simulink model "qarm_quick_start_model_virtual"  (R2020a)
settings: Solver=ode4  StartTime=0.0  StopTime=Inf  FixedStep=1/500  RelTol=1e-3
undefined symbols (not defined in the file): HIL
libraries: quarc_library x7, simulink_extras x2
settings Model: ExtModeTrigDuration=10000  Creator=fvranes  LastModifiedBy=mbohra
settings DebuggingCC: UnderspecifiedInitializationDetection=Classic  MergeDetectMultiDrivingBlocksExec=none
settings ModelReferenceCC: PropagateSignalLabelsOutOfModel=off
settings SFSimCC: CustomCodeUndefinedFunction=UseInterfaceOnly

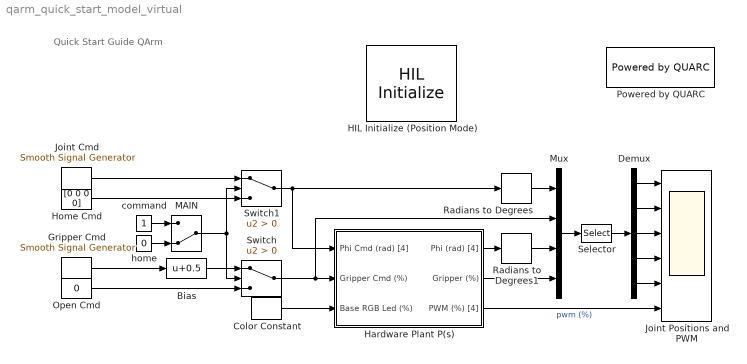
== system qarm_quick_start_model_virtual ==
  note: Quick Start Guide
      | QArm
  Bias : Bias  Bias=0.5
  Color Constant : quarc_library/Sources/Signals/Color Constant  color=[0 1 0]
      settings: SourceProductName=QUARC Targets
  Demux : Demux  Outputs=[2 2 2 2 2]
  Gripper Cmd : quarc_library/Sources/Signals/Smooth Signal Generator  signal_type=Square  source=Internal (dialog parameters)  amplitude=0.5  frequency=0.25  initial_phase=0  sample_time=qc_get_step_size  output_cos=off
      settings: SourceProductName=QUARC Targets
  HIL Initialize (Position Mode) : quarc_library/Data Acquisition/Generic/Configuration/HIL Initialize  object_name=HIL-1  board_type=qarm_usb  board_number=0@tcpip://localhost:18900?nagle='off'  board_options=j0_mode=0;j1_mode=0;j2_mode=0;j3_mode=0;gripper_mode=0;  exclusive=off  active=on  hardware_clocks=[0]  clock_modes=[]  initial_clock_frequencies=[]  set_clock_params_at_start=off  set_clock_params_at_switch_in=off  set_clock_frequencies_at_start=off  set_clock_frequencies_at_switch_in=off  analog_input_channels=[5:9]  analog_input_configurations=[]  analog_input_maximums=[]  analog_input_minimums=[]  set_analog_input_params_at_start=off  set_analog_input_params_at_switch_in=off  analog_output_channels=[]  analog_output_maximums=inf  analog_output_minimums=-inf  initial_analog_outputs=[0]  final_analog_outputs=[0]  watchdog_analog_outputs=[]  set_analog_output_params_at_start=off  set_analog_output_params_at_switch_in=off  set_analog_outputs_at_start=off  set_analog_outputs_at_switch_in=off  set_analog_outputs_at_terminate=off  set_analog_outputs_at_switch_out=off  set_analog_outputs_on_watchdog=off  digital_input_channels=[]  digital_output_channels=[]  digital_output_configuration=[]  initial_digital_outputs=[0]  final_digital_outputs=[0]  watchdog_digital_outputs=[0]  set_digital_output_params_at_start=off  set_digital_output_params_at_switch_in=off  set_digital_outputs_at_start=off  set_digital_outputs_at_switch_in=off  set_digital_outputs_at_terminate=off  set_digital_outputs_at_switch_out=off  set_digital_outputs_on_watchdog=off  encoder_channels=[]  quadrature=[]  encoder_filter_frequency=[]  initial_encoder_counts=[]  set_encoder_params_at_start=off  set_encoder_params_at_switch_in=off  set_encoder_counts_at_start=off  set_encoder_counts_at_switch_in=off  pwm_channels=[]  pwm_modes=[]  pwm_frequency=[]  pwm_configuration=[]  pwm_alignment=[]  pwm_polarity=[]  pwm_leading_deadband=[]  pwm_trailing_deadband=[]  initial_pwm_outputs=[]  final_pwm_outputs=[]  watchdog_pwm_outputs=[]  set_pwm_params_at_start=off  set_pwm_params_at_switch_in=off  set_pwm_outputs_at_start=off  set_pwm_outputs_at_switch_in=off  set_pwm_outputs_at_terminate=off  set_pwm_outputs_at_switch_out=off  set_pwm_outputs_on_watchdog=off  other_output_channels=[1000:1004 11000:11003 11005:11007]  initial_other_outputs=[zeros(1,9), ones(1,3)]  final_other_outputs=[zeros(1,9), ones(1,3)]  watchdog_other_outputs=zeros(1,12)  set_other_outputs_at_start=off  set_other_outputs_at_switch_in=off  set_other_outputs_at_terminate=on  set_other_outputs_at_switch_out=off  set_other_outputs_on_watchdog=off
  Hardware Plant P(s) : Subsystem
  Home Cmd : Constant  Value=[0 0 0 0]
  Joint Cmd : quarc_library/Sources/Signals/Smooth Signal Generator  signal_type=Square  source=Internal (dialog parameters)  amplitude=[pi/8 pi/8 pi/8 pi/8]  frequency=0.25  initial_phase=[0 0 pi 0]  sample_time=qc_get_step_size  output_cos=off
      settings: SourceProductName=QUARC Targets
  Joint Positions and PWM : Scope  NumInputPorts=6
  MAIN : ManualSwitch  CurrentSetting=0
  Mux : Mux
  Open Cmd : Constant  Value=0
  Powered by QUARC : quarc_library/Logos/Powered by QUARC
  Radians to Degrees : simulink_extras/Transformations/Radians to Degrees
  Radians to Degrees1 : simulink_extras/Transformations/Radians to Degrees
  Selector : Selector  InputPortWidth=10  IndexOptions=Index vector (dialog)  Indices=[1 6 2 7 3 8 4 9 5 10]  OutputSizes=1
  Switch : Switch  Criteria=u2 > Threshold
  Switch1 : Switch  Criteria=u2 > Threshold
  command : Constant
  home : Constant  Value=0
  wires:
  Color Constant/1 -> Hardware Plant P(s)/3(Base RGB Led (%))
  Switch/1 -> Mux/2, Hardware Plant P(s)/2(Gripper Cmd (%))
  Home Cmd/1 -> Switch1/3
  Joint Cmd/1 -> Switch1/1
  Switch1/1 -> Radians to Degrees/1, Hardware Plant P(s)/1(Phi Cmd (rad) [4])
  Hardware Plant P(s)/1(Phi (rad) [4]) -> Radians to Degrees1/1
  Hardware Plant P(s)/2(Gripper (%)) -> Mux/4
  Mux/1 -> Selector/1
  Hardware Plant P(s)/3(PWM (%) [4]) -> Joint Positions and PWM/6  "pwm (%)"
  Radians to Degrees/1 -> Mux/1
  Radians to Degrees1/1 -> Mux/3
  Selector/1 -> Demux/1
  Demux/1 -> Joint Positions and PWM/1
  Demux/2 -> Joint Positions and PWM/2
  Demux/3 -> Joint Positions and PWM/3
  Demux/4 -> Joint Positions and PWM/4
  Demux/5 -> Joint Positions and PWM/5
  Open Cmd/1 -> Switch/3
  Gripper Cmd/1 -> Bias/1
  MAIN/1 -> Switch/2, Switch1/2
  home/1 -> MAIN/2
  command/1 -> MAIN/1
  Bias/1 -> Switch/1

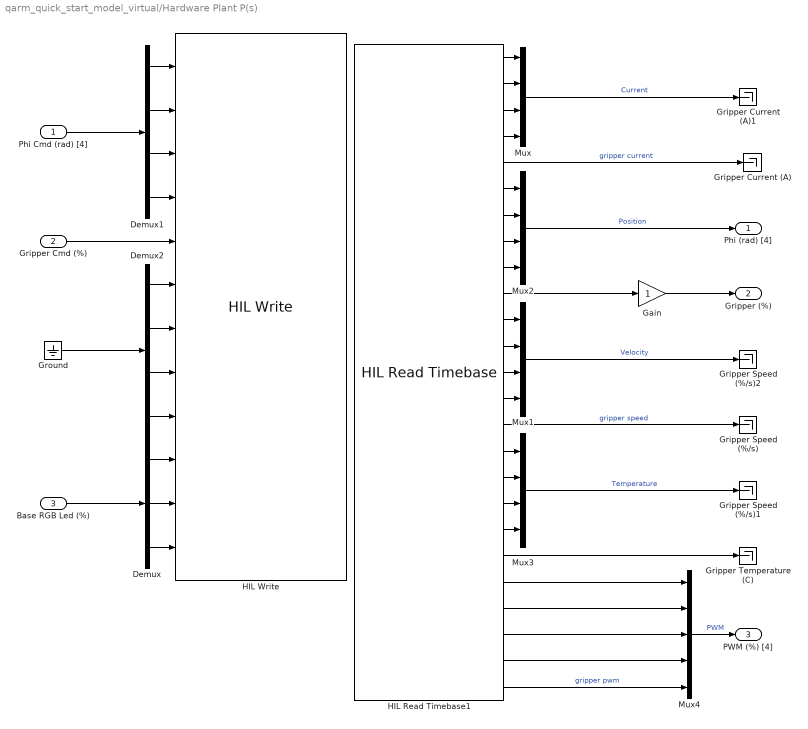
== system qarm_quick_start_model_virtual/Hardware Plant P(s) ==
  Phi Cmd (rad) [4] : Inport
  Gripper Cmd (%) : Inport  Port=2
  Base RGB Led (%) : Inport  Port=3
  Demux : Demux  Outputs=3
  Demux1 : Demux
  Demux2 : Demux
  Gain : Gain
  Gripper Current (A) : Terminator
  Gripper Current (A)1 : Terminator
  Gripper Speed (%/s) : Terminator
  Gripper Speed (%/s)1 : Terminator
  Gripper Speed (%/s)2 : Terminator
  Gripper Temperature (C) : Terminator
  Ground : Ground
  HIL Read Timebase1 : quarc_library/Data Acquisition/Generic/Timebases/HIL Read Timebase  object_name=HIL-1  clock=0  analog_channels=[5:9]  encoder_channels=[]  digital_channels=[]  other_channels=[1000:1004 3000:3004 10000:10004 11000:11004]  active=on  vector_output=off  data_type_mode=Inherit via back propagation  encoder_data_type=double  digital_data_type=boolean  overflow_mode=Synchronize (for simulated cards only)  samples_in_buffer=1
  HIL Write : quarc_library/Data Acquisition/Generic/Immediate I//O/HIL Write  object_name=HIL-1  analog_channels=[]  pwm_channels=[]  digital_channels=[]  other_channels=[1000:1004 11000:11003 11005:11007]  sample_time=-1  active=on  vector_input=off
  Mux{,1..3} (4 alike) : Mux
  Mux4 : Mux  Inputs=5
  Phi (rad) [4] : Outport  VectorParamsAs1DForOutWhenUnconnected=off
  Gripper (%) : Outport  Port=2  VectorParamsAs1DForOutWhenUnconnected=off
  PWM (%) [4] : Outport  Port=3  VectorParamsAs1DForOutWhenUnconnected=off
  wires:
  Gripper Cmd (%)/1 -> HIL Write/5
  Gain/1 -> Gripper (%)/1
  HIL Read Timebase1/10 -> Gain/1
  Mux4/1 -> PWM (%) [4]/1  "PWM"
  HIL Read Timebase1/25 -> Mux4/5  "gripper pwm"
  HIL Read Timebase1/24 -> Mux4/4
  HIL Read Timebase1/23 -> Mux4/3
  HIL Read Timebase1/22 -> Mux4/2
  HIL Read Timebase1/21 -> Mux4/1
  Mux2/1 -> Phi (rad) [4]/1  "Position"
  Demux2/4 -> HIL Write/9
  Demux2/3 -> HIL Write/8
  Demux2/2 -> HIL Write/7
  Demux2/1 -> HIL Write/6
  Ground/1 -> Demux2/1
  Phi Cmd (rad) [4]/1 -> Demux1/1
  Demux1/4 -> HIL Write/4
  Demux1/3 -> HIL Write/3
  Demux1/2 -> HIL Write/2
  Demux1/1 -> HIL Write/1
  Base RGB Led (%)/1 -> Demux/1
  Mux3/1 -> Gripper Speed (%/s)1/1  "Temperature"
  Mux1/1 -> Gripper Speed (%/s)2/1  "Velocity"
  Mux/1 -> Gripper Current (A)1/1  "Current"
  HIL Read Timebase1/20 -> Gripper Temperature (C)/1
  HIL Read Timebase1/1 -> Mux/1
  HIL Read Timebase1/2 -> Mux/2
  HIL Read Timebase1/13 -> Mux1/3
  Demux/2 -> HIL Write/11
  HIL Read Timebase1/19 -> Mux3/4
  Demux/1 -> HIL Write/10
  HIL Read Timebase1/11 -> Mux1/1
  HIL Read Timebase1/16 -> Mux3/1
  HIL Read Timebase1/17 -> Mux3/2
  HIL Read Timebase1/3 -> Mux/3
  Demux/3 -> HIL Write/12
  HIL Read Timebase1/15 -> Gripper Speed (%/s)/1  "gripper speed"
  HIL Read Timebase1/5 -> Gripper Current (A)/1  "gripper current"
  HIL Read Timebase1/7 -> Mux2/2
  HIL Read Timebase1/4 -> Mux/4
  HIL Read Timebase1/12 -> Mux1/2
  HIL Read Timebase1/8 -> Mux2/3
  HIL Read Timebase1/18 -> Mux3/3
  HIL Read Timebase1/6 -> Mux2/1
  HIL Read Timebase1/9 -> Mux2/4
  HIL Read Timebase1/14 -> Mux1/4
